simulink model "example"  (R2023a)
settings: Solver=FixedStepAuto  StartTime=0.0  StopTime=inf  RelTol=1e-3
libraries: mttlib x7, instrumentseriallib x1
settings Model: Creator=chrismailer  LastModifiedBy=JesseJabezArendse
settings DebuggingCC: ParameterPrecisionLossMsg=none
settings ModelReferenceCC: EnableRefExpFcnMdlSchedulingChecks=on
settings SFSimCC: SimTargetLang=C++

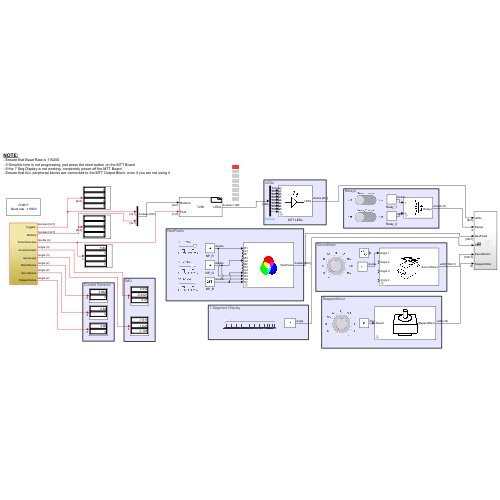
[thumbnail: Simulink's stored preview of the top-level diagram]
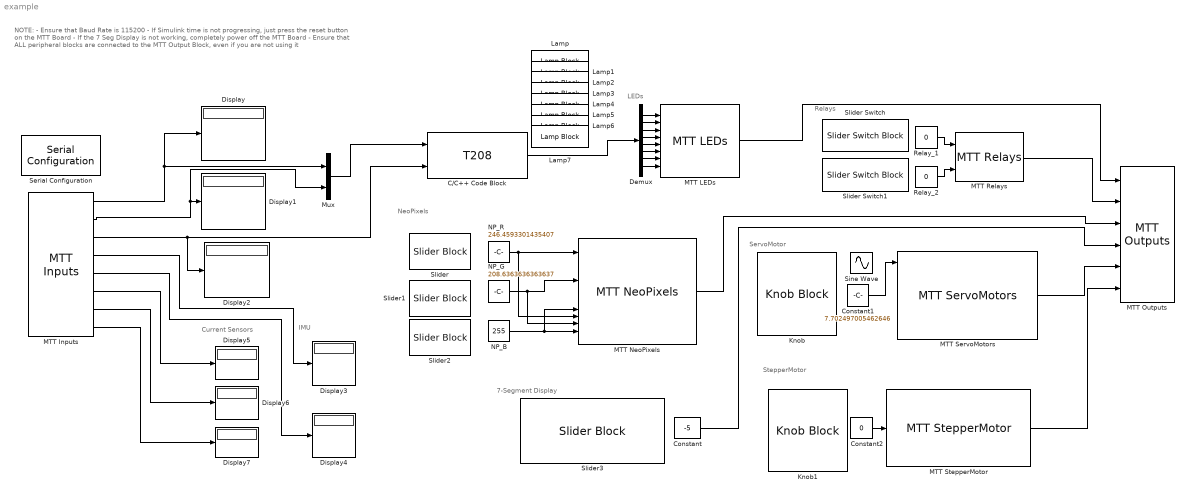
== system example ==
  note: Current Sensors
  note: NOTE:
      | - Ensure that Baud Rate is 115200
      | - If Simulink time is not progressing, just press the reset button on the MTT Board
      | - If the 7 Seg Display is not working, completely power off the MTT Board
      | - Ensure that ALL peripheral blocks are connected to the MTT Output Block, even if you are not using it
  note: IMU
  note: 7-Segment Display
  note: ServoMotor
  note: StepperMotor
  note: LEDs
  note: NeoPixels
  note: Relays
  C/C++ Code Block : S-Function  FunctionName=T208  SFunctionModules=T208_wrapper.cpp  SFunctionDeploymentMode=off  EnableBusSupport=off  mask(S-Function Builder){}
      mask help: Simulink:masks:SFunctionBuilder_MD
      mask init:
      | val = [[.9  0.75 0.75 1 1 .9 .9 1]',[1 1 0.75 0.75 .9 .9 1 .9]'];try , sys = get_param(gcb,'SfunBuilderFcnName');if isempty(sys), sys = get_param(gcb,'FunctionName'); end,catch, sys = get_param(gcb,'FunctionName'); end
      settings: CopyFcn=set_param(gcbh,'LinkStatus','none')  OpenFcn=sfunctionwizard(gcbh)
      mask Display:
      | plot(val(:,1),val(:,2))
      | disp(sys)
      | port_label('input',1,'Buttons')
      | port_label('input',2,'Pots')
      | port_label('output',1,'LEDs')
  Constant : Constant  Value=-5  OutDataTypeStr=single
  Constant1 : Constant  Value=7.702497005462646
  Constant2 : Constant  Value=0
  Demux : Demux  Outputs=8
  Display{,1..7} (8 alike) : Display
  Knob : KnobBlock  LabelPosition=Hide  ScaleMax=150
  Knob1 : KnobBlock  LabelPosition=Hide  ScaleMax=1
  Lamp{,1..7} (8 alike) : LampBlock  LabelPosition=Hide  Icon=Rectangle
  MTT Inputs : mttlib/MTT Inputs  SystemSampleTime=-1  VariantActivationTime=update diagram  Latency=0  AutoFrameSizeCalculation=off
      settings: SourceProductName=MTT Library
  MTT LEDs : mttlib/MTT LEDs
      settings: SourceProductName=MTT Library
  MTT NeoPixels : mttlib/MTT NeoPixels
      settings: SourceProductName=MTT Library
  MTT Outputs : mttlib/MTT Outputs  SystemSampleTime=-1  VariantActivationTime=update diagram  Latency=0  AutoFrameSizeCalculation=off
      settings: SourceProductName=MTT Library
  MTT Relays : mttlib/MTT Relays
      settings: SourceProductName=MTT Library
  MTT ServoMotors : mttlib/MTT ServoMotors  maxAngle1=150  startingTime1=100  maxAngle2=0  startingTime2=0  maxAngle3=0  startingTime3=0  maxAngle4=0  startingTime4=0
      settings: SourceProductName=MTT Library
  MTT StepperMotor : mttlib/MTT StepperMotor  stepperMode=Half  stepperRevolution=1024
      settings: SourceProductName=MTT Library
  Mux : Mux  Inputs=2
  NP_B : Constant  Value=255
  NP_G : Constant  Value=208.6363636363637
  NP_R : Constant  Value=246.4593301435407
  Relay_1 : Constant  Value=0
  Relay_2 : Constant  Value=0
  Serial Configuration : instrumentseriallib/Serial Configuration  Priority=-200000  PortSel=COM17  Port=COM17  ComPort=COM17  BaudRate=115200  DataBits=8  Parity=none  StopBits=1  ByteOrder=little-endian  FlowControl=none  Timeout=100  SimulateUsing=Interpreted execution  BlockInModel=on  aMode=1
      settings: LibrarySourceBlock=embeddedtargetslib/Host Communication/Serial Configuration
  Sine Wave : Sin  Amplitude=45  Bias=45  Frequency=15  SampleTime=0
  Slider : SliderBlock  ScaleMax=255
  Slider Switch : SliderSwitchBlock
      settings: Values={{'Off', 'On'}, [0 1]}
  Slider Switch1 : SliderSwitchBlock
      settings: Values={{'Off', 'On'}, [0 1]}
  Slider1 : SliderBlock  ScaleMax=255
  Slider2 : SliderBlock  ScaleMax=255
  Slider3 : SliderBlock  LabelPosition=Hide  ScaleMin=-5  ScaleMax=5  TickInterval=0.1
  wires:
  Relay_1/1 -> MTT Relays/1
  Relay_2/1 -> MTT Relays/2
  MTT Inputs/1 -> Display/1, Mux/1
  MTT Inputs/2 -> Mux/2, Display1/1
  MTT Inputs/3 -> Display2/1, C/C++ Code Block/2
  MTT Inputs/4 -> Display3/1
  MTT Inputs/5 -> Display4/1
  Constant2/1 -> MTT StepperMotor/1
  NP_R/1 -> MTT NeoPixels/10, MTT NeoPixels/1
  NP_G/1 -> MTT NeoPixels/11, MTT NeoPixels/5
  NP_B/1 -> MTT NeoPixels/12, MTT NeoPixels/9
  MTT Inputs/6 -> Display5/1
  MTT Inputs/7 -> Display6/1
  MTT Inputs/8 -> Display7/1
  MTT LEDs/1 -> MTT Outputs/1
  Constant/1 -> MTT Outputs/4
  MTT Relays/1 -> MTT Outputs/2
  MTT NeoPixels/1 -> MTT Outputs/3
  MTT ServoMotors/1 -> MTT Outputs/5
  MTT StepperMotor/1 -> MTT Outputs/6
  Constant1/1 -> MTT ServoMotors/1
  Demux/1 -> MTT LEDs/1
  Demux/2 -> MTT LEDs/2
  Demux/3 -> MTT LEDs/3
  Demux/4 -> MTT LEDs/4
  Demux/5 -> MTT LEDs/5
  Demux/6 -> MTT LEDs/6
  Demux/7 -> MTT LEDs/7
  Demux/8 -> MTT LEDs/8
  C/C++ Code Block/1 -> Demux/1
  Mux/1 -> C/C++ Code Block/1
